simulink model "dcmotor"  (R2021a)
settings: Solver=VariableStepAuto  StartTime=0.0  StopTime=100  RelTol=1e-3
settings Model: Creator=SREETAM  LastModifiedBy=SREETAM

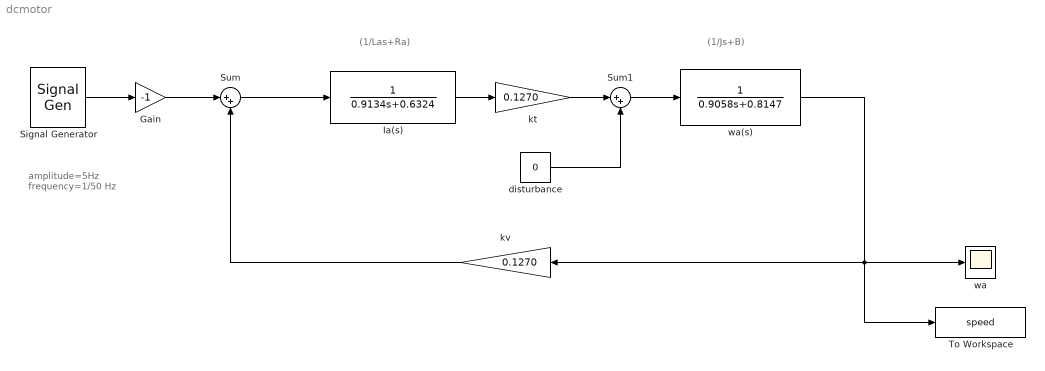
== system dcmotor ==
  note: amplitude=5Hz
      | frequency=1/50 Hz
  note: (1/Las+Ra)
  note: (1/Js+B)
  Gain : Gain  Gain=-1
  Ia(s) : TransferFcn  Denominator=[0.9134 0.6324]
  Signal Generator : SignalGenerator  WaveForm=square  Amplitude=5  Frequency=1/50
  Sum : Sum  Inputs=|++
  Sum1 : Sum  Inputs=|++
  To Workspace : ToWorkspace  VariableName=speed  SaveFormat=Timeseries  SampleTime=-1
  disturbance : Constant  Value=0
  kt : Gain  Gain=0.1270
  kv : Gain  Gain=0.1270
  wa : Scope
  "wa(s) " : TransferFcn  Denominator=[0.9058 0.8147]
  wires:
  Ia(s)/1 -> kt/1
  Sum/1 -> Ia(s)/1
  Sum1/1 -> "wa(s) "/1
  Signal Generator/1 -> Gain/1
  Gain/1 -> Sum/1
  kt/1 -> Sum1/1
  disturbance/1 -> Sum1/2
  kv/1 -> Sum/2
  "wa(s) "/1 -> To Workspace/1, kv/1, wa/1
